simulink model "g_Inverse_Dynamic"  (R2015a)
settings: Solver=ode2  StartTime=0.0  StopTime=10.0  FixedStep=0.01  RelTol=1e-3
InitFcn:
  | Parameters
values from neighbouring files (symbols this model uses):
  Kinv = K\eye(4)    [Parameters.m]    (also in Parameters_controllers.m = [ -1/(4*Kt),  2^(1/2)/(4*Kt*b),  2^(1/2)/(4*Kt*b), -1/(4*Kq))
  x1 = [m q]    [Parameters.m]
settings Model: Creator=pela  LastModifiedBy=pela
settings HardwareCC: ProdLargestAtomicInteger=Long  ProdLargestAtomicFloat=Double  ProdEndianess=LittleEndian  ProdHWDeviceType=ARM Compatible->ARM Cortex
settings RTWCC: GenCodeOnly=on  GenerateReport=on  BuildConfiguration=Faster Runs  LaunchReport=on  TargetLang=C++
settings GRTTargetCC: MatFileLogging=off  MultiInstanceERTCode=on  CodeInterfacePackaging=C++ class

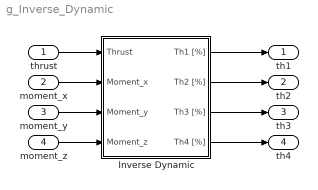
== system g_Inverse_Dynamic ==
  thrust : Inport
  moment_x : Inport  Port=2
  moment_y : Inport  Port=3
  moment_z : Inport  Port=4
  Inverse Dynamic : Subsystem  InitFcn=|
      | %%Parameters definition
      | b = 0.55/2;
      | RPMmax = 3*4.2*710;
      | D = 12*2.54/100;
      | Ct = 0.001;
      | Cq = 0.001;
      | ro = 1.225;
      | 
      | %% From omega squared to forces/torques
      |  A = ro*D^4*diag([Ct b/sqrt(2)*Ct b/sqrt(2)*Ct Cq*D]);
      |  B = [ 1  1  1 1;
      |          1 -1 -1 1;
      |         -1 -1  1 1;
      |         -1  1 -1 1];
      |  C = inv(A*B);       %TM = C * omegasq
  th1 : Outport
  th2 : Outport  Port=2
  th3 : Outport  Port=3
  "th4 " : Outport  Port=4
  wires:
  thrust/1 -> Inverse Dynamic/1(Thrust)
  moment_x/1 -> Inverse Dynamic/2(Moment_x)
  moment_y/1 -> Inverse Dynamic/3(Moment_y)
  moment_z/1 -> Inverse Dynamic/4(Moment_z)
  Inverse Dynamic/4(Th4 [%]) -> "th4 "/1
  Inverse Dynamic/3(Th3 [%]) -> th3/1
  Inverse Dynamic/2(Th2 [%]) -> th2/1
  Inverse Dynamic/1(Th1 [%]) -> th1/1

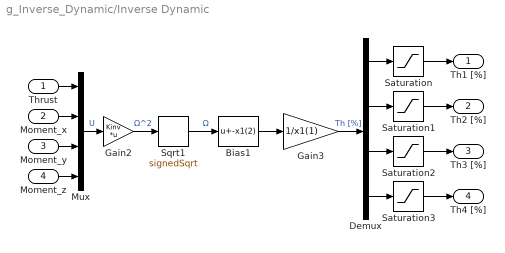
== system g_Inverse_Dynamic/Inverse Dynamic ==
  Thrust : Inport
  Moment_x : Inport  Port=2
  Moment_y : Inport  Port=3
  Moment_z : Inport  Port=4
  Bias1 : Bias  Bias=-x1(2)
  Demux : Demux
  Gain2 : Gain  Gain=Kinv  Multiplication=Matrix(K*u)
  Gain3 : Gain  Gain=1/x1(1)
  Mux : Mux
  Saturation{,1..3} (4 alike) : Saturate  UpperLimit=100  LowerLimit=0
  Sqrt1 : Sqrt  Operator=signedSqrt  SaturateOnIntegerOverflow=on
  Th1 [%] : Outport
  Th2 [%] : Outport  Port=2
  Th3 [%] : Outport  Port=3
  Th4 [%] : Outport  Port=4
  wires:
  Thrust/1 -> Mux/1
  Moment_z/1 -> Mux/4
  Moment_y/1 -> Mux/3
  Moment_x/1 -> Mux/2
  Demux/1 -> Saturation/1
  Saturation/1 -> Th1 [%]/1
  Demux/2 -> Saturation1/1
  Demux/3 -> Saturation2/1
  Demux/4 -> Saturation3/1
  Saturation3/1 -> Th4 [%]/1
  Saturation2/1 -> Th3 [%]/1
  Saturation1/1 -> Th2 [%]/1
  Gain3/1 -> Demux/1  "Th [%]"
  Bias1/1 -> Gain3/1
  Gain2/1 -> Sqrt1/1  "Ω^2"
  Mux/1 -> Gain2/1  "U"
  Sqrt1/1 -> Bias1/1  "Ω"
